simulink library "calcGravForce_ul"  (R2020a)
settings: Solver=VariableStepAuto  StartTime=0.0  StopTime=10.0  RelTol=1e-3
settings Model: Creator=Ayaz  LastModifiedBy=Ayaz

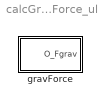
== system calcGravForce_ul ==
  gravForce : Subsystem  mask{gravAccl=9.81, mKite=36}
      mask prompts: gravAccl "Gravitational accleration [m/s^2]"; mKite "Kite mass [kg]"
      mask TypeOptions gravAccl: Constant1/Value
      mask TypeOptions mKite: Constant2/Value

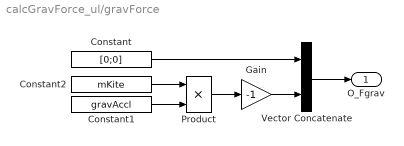
== system calcGravForce_ul/gravForce ==
  Constant : Constant  Value=[0;0]
  Constant1 : Constant  Value=gravAccl
  Constant2 : Constant  Value=mKite
  Gain : Gain  Gain=-1
  Product : Product
  Vector Concatenate : Concatenate
  O_Fgrav : Outport  PortDimensions=[3,1]
  wires:
  Constant2/1 -> Product/1
  Constant1/1 -> Product/2
  Product/1 -> Gain/1
  Constant/1 -> Vector Concatenate/1
  Vector Concatenate/1 -> O_Fgrav/1
  Gain/1 -> Vector Concatenate/2
